simulink model "testScript_model_EGC"  (Simulink 8.1)
settings: Solver=ode3  SolverMode=SingleTasking  StartTime=0.0  StopTime=20000  FixedStep=Ts  RelTol=1e-3
PostLoadFcn:
  | Ts=1;
InitFcn:
  | Ts=1;
values from neighbouring files (symbols this model uses):
  CMD_signals = [0 300 600 900 1200 1500 1800 2100 2400 2700 3000 3300 ... (1568 elements, 49x32)]    [CMD_signals.mat]
libraries: artemis x1, rtio_generic_modbus x1, powerlib x1
settings Model: ARTEMISmethode_block_infos=$$__separator__$$testScript_model_EGC/ARTEMIS Guide$$__separator__$$  Creator=ma25949  LastModifiedBy=ed12083
settings OptimizationCC: BlockReduction=off  BooleanDataType=off  ExpressionDepthLimit=128
settings DebuggingCC: SaveWithParameterizedLinksMsg=none  SignalResolutionControl=TryResolveAllWithWarning  SolverPrmCheckMsg=none  MultiTaskDSMMsg=warning  MultiTaskCondExecSysMsg=none  FcnCallInpInsideContextMsg=EnableAllAsError  StrictBusMsg=None
settings HardwareCC: TargetUnknown=on
settings RTWCC: IncludeERTFirstTime=on
settings GRTTargetCC: CombineOutputUpdateFcns=on  GRTInterface=off

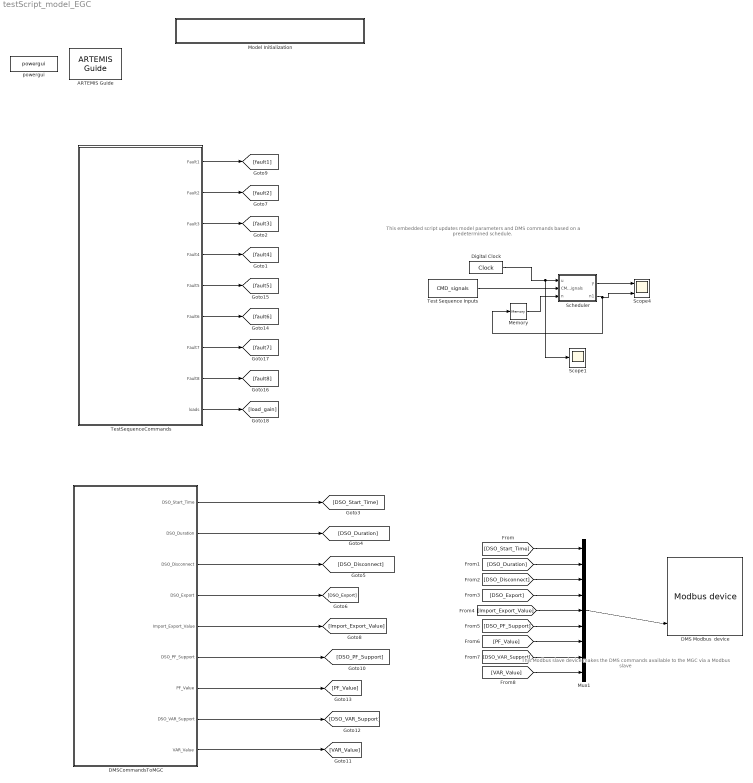
== system testScript_model_EGC ==
  note: This Modbus slave device makes the DMS
      | commands available to the MGC via a Modbus
      | slave
  note: This embedded script updates model
      | parameters and DMS commands based
      | on a predetermined schedule.
  ARTEMIS Guide : artemis/ARTEMIS/ARTEMIS Guide  Tag=FTSSmethode_opal_4hx0r99  Description=5.0_z1  lock=on  Ts=Ts  opt=art5  dyna=off  nb_perm=4  RT_fullcomp=off  ssn=on  ssn_itvc=off  ssn_ivic=off  ssn_ext=off  ssn_solver=Art5 with Backward Euler nodal interface  ssn_impulse=off  ssn_quasimpulse=off  ssn_impulse_loop=2  paraExtinctionThy=off  Thy_Impulse=on  dtc=Off  dtc_opt=normal  ao=on  simtype=off  ct_mac=off  lin_mov=off  lsp=[0.001 2]  spike_skip=Disabled  dtc_extra=1  dtc_sws=normal  dtc_pied=0.5  SPSRulesBlock=SPSRules  tre=on  ctmm=off  LF=off  dpl_type=ARTEMiS DPL  rlc_type=off  custom_type=off  para=on  ssn_ImpulseLoopBlockedStateUpdate=2  ssn_mov_iter_number=5  ssn_switch_iter_number=5
  DMS Modbus  device : rtio_generic_modbus/Modbus device  conf_name=DMS_slave_cfg.opal  conf_name_mask=DMS_slave_cfg.xls  sample_time=0
  DMSCommandsToMGC : Subsystem  mask{DSO_Start_Time=0, DSO_Duration=0, DSO_Disconnect=0, DSO_Export=0, Import_Export_Value=0, DSO_PF_Support=0, PF_Value=0, DSO_VAR_Support=0, VAR_Value=1000}
      mask prompts: DSO_Start_Time "DSO Start Time"; DSO_Duration "DSO Duration"; DSO_Disconnect "DSO Disconnect"; DSO_Export "DSO Export (1) or Import (0)"; Import_Export_Value "Import/Export Value, kW"; DSO_PF_Support "DSO PF Support (1) or Not (0)"; PF_Value "PF Value, pu, "+"(lagging) "-" (leading)"; DSO_VAR_Support "DSO VAR Support (1) or Not (0)"; VAR_Value "Import/Export Value, kVAr"
  Digital Clock : DigitalClock  SampleTime=Ts
  Memory : Memory  X0=1
  Model Initialization : Subsystem  AncestorBlock=artemis/Tools /Misc/Model Initialization  mask(Model Functions){InitFcnX=Ts=1;, prel=off, posl=on, inif=on, strf=off}
      mask prompts: InitFcnX "Initialisation"; prel "Preload Function"; posl "PostLoad Function"; inif "InitFcn"; strf "StartFcn"
      mask init:
      | currentBlock = gcb;
      | root = bdroot(currentBlock);
      | 
      | 
      | if ~strcmp(get_param(root,'BlockDiagramType'),'library')
      |     if prel==1
      |         set_param(root, 'PreLoadFcn', InitFcnX);
      |     else
      |         set_param(root, 'PreLoadFcn', '');
      |     end
      |     if inif==1
      |         set_param(root, 'InitFcn', InitFcnX);
      |     else
      |         set_param(root, 'InitFcn', '');
      |     end
      |     if strf==1
      |         set_param(root, 'StartFcn', InitFcnX);
      |     else
      |         set_param(root, 'StartFcn', '');
      |     end
      |     if posl==1
      |         set_param(root, 'PostLoadFcn', InitFcnX);
      |     else
      |         set_param(root, 'PostLoadFcn', '');
      |     end
      | end
      | 
      | pos = get_param(currentBlock, 'Position');
      | width = pos(3) - pos(1); height = pos(4) - pos(2);
      | txt = [ upper(root) '\n' '- InitFcn. . . . . '  get_param(root, 'InitFcn') ];
      settings: CopyFcn=set_param(gcb,'LinkStatus','inactive')
      mask Display: text(5, height*0.5, txt, 'horizontalAlignment', 'left', 'verticalAlignment', 'middle') ;
  Mux1 : Mux  Inputs=9
  Scheduler : MATLAB Function  TreatAsAtomicUnit=on
  Scope1 : Scope
      settings: YMin=1.04083e-17  YMax=0.2  SaveName=ScopeData4
  Scope4 : Scope  NumInputPorts=3
      settings: YMin=-5~-5~-5  YMax=5~5~5
  Test Sequence Inputs : Constant  Value=CMD_signals
  TestSequenceCommands : Subsystem  mask{fault1=0, fault2=0, fault3=0, fault4=0, fault5=0, fault6=0, fault7=0, fault8=0, load_gain=1}
      mask prompts: load_gain "Loads"
  powergui : powerlib/powergui  Priority=2  SimulationMode=Discrete  SolverType=Tustin  SampleTime=Ts  frequency=60  SPID=off  DisableSnubberDevices=off  DisableRonSwitches=off  DisableVfSwitches=off  SwTol=0  Interpol=off  DisplayEquations=off  frequencyindice=0  Pbase=100e6  ErrMax=1e-4  Iterations=50  UnitsV=kV  UnitsW=MW  FunctionMessages=off  echomessages=off  HookPort=off  EnableUseOfTLC=off  x0status=blocks  RestoreLinks=warning  ResistiveCurrentMeasurement=off  Frange=logspace(0,3,50)  Ylog=off  Xlog=off  ShowGrid=off  save=off  variable=ZData  structure=0  ZoomFFT=on  StartTime=0.0  cycles=2  DisplayStyle=off  fundamental=60  FreqAxis=off  MaxFrequency=1000  frequencyindicesteady=1  RmsSteady=1  display=off  Ts=0  methode=off
  wires:
  Mux1/1 -> DMS Modbus  device/4
  Scheduler/1(y) -> Scope4/1
  Scheduler/2(n1) -> Scope4/3, Memory/1
  Memory/1 -> Scheduler/3(n)
  Test Sequence Inputs/1 -> Scheduler/2(CMD_signals)
  Digital Clock/1 -> Scope1/1, Scheduler/1(u)
  DMSCommandsToMGC/3(DSO_Disconnect) -> [DSO_Disconnect]
  DMSCommandsToMGC/4(DSO_Export) -> [DSO_Export]
  DMSCommandsToMGC/6(DSO_PF_Support) -> [DSO_PF_Support]
  DMSCommandsToMGC/8(DSO_VAR_Support) -> [DSO_VAR_Support]
  DMSCommandsToMGC/9(VAR_Value) -> [VAR_Value]
  DMSCommandsToMGC/7(PF_Value) -> [PF_Value]
  DMSCommandsToMGC/1(DSO_Start_Time) -> [DSO_Start_Time]
  DMSCommandsToMGC/2(DSO_Duration) -> [DSO_Duration]
  DMSCommandsToMGC/5(Import_Export_Value) -> [Import_Export_Value]
  [DSO_Start_Time] -> Mux1/1
  [DSO_Duration] -> Mux1/2
  [DSO_Disconnect] -> Mux1/3
  [DSO_Export] -> Mux1/4
  [Import_Export_Value] -> Mux1/5
  [DSO_PF_Support] -> Mux1/6
  [PF_Value] -> Mux1/7
  [DSO_VAR_Support] -> Mux1/8
  [VAR_Value] -> Mux1/9
  TestSequenceCommands/1(Fault1) -> [fault1]
  TestSequenceCommands/2(Fault2) -> [fault2]
  TestSequenceCommands/3(Fault3) -> [fault3]
  TestSequenceCommands/4(Fault4) -> [fault4]
  TestSequenceCommands/5(Fault5) -> [fault5]
  TestSequenceCommands/6(Fault6) -> [fault6]
  TestSequenceCommands/7(Fault7) -> [fault7]
  TestSequenceCommands/8("Fault8 ") -> [fault8]
  TestSequenceCommands/9(loads) -> [load_gain]

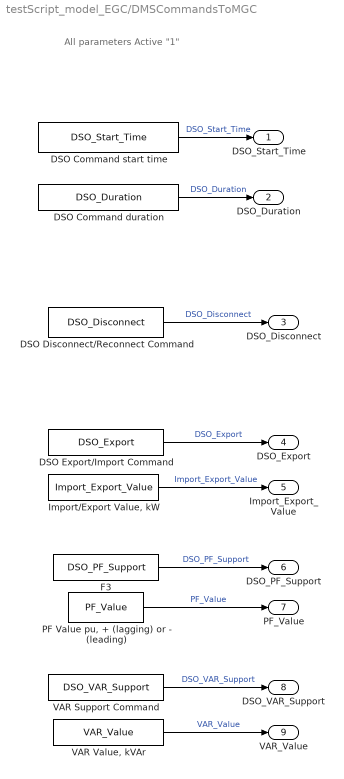
== system testScript_model_EGC/DMSCommandsToMGC ==
  note: All parameters Active "1"
  DSO Command duration : Constant  Value=DSO_Duration
  DSO Command start time : Constant  Value=DSO_Start_Time
  DSO Disconnect/Reconnect Command : Constant  Value=DSO_Disconnect
  DSO Export/Import Command : Constant  Value=DSO_Export
  F3 : Constant  Value=DSO_PF_Support
  "Import/Export Value, kW" : Constant  Value=Import_Export_Value
  "PF Value pu, + (lagging) or - (leading)" : Constant  Value=PF_Value
  VAR Support Command : Constant  Value=DSO_VAR_Support
  "VAR Value, kVAr" : Constant  Value=VAR_Value
  DSO_Start_Time : Outport
  DSO_Duration : Outport  Port=2
  DSO_Disconnect : Outport  Port=3
  DSO_Export : Outport  Port=4
  Import_Export_Value : Outport  Port=5
  DSO_PF_Support : Outport  Port=6
  PF_Value : Outport  Port=7
  DSO_VAR_Support : Outport  Port=8
  VAR_Value : Outport  Port=9
  wires:
  DSO Disconnect/Reconnect Command/1 -> DSO_Disconnect/1  "DSO_Disconnect"
  DSO Export/Import Command/1 -> DSO_Export/1  "DSO_Export"
  F3/1 -> DSO_PF_Support/1  "DSO_PF_Support"
  VAR Support Command/1 -> DSO_VAR_Support/1  "DSO_VAR_Support"
  "VAR Value, kVAr"/1 -> VAR_Value/1  "VAR_Value"
  "PF Value pu, + (lagging) or - (leading)"/1 -> PF_Value/1  "PF_Value"
  DSO Command start time/1 -> DSO_Start_Time/1  "DSO_Start_Time"
  DSO Command duration/1 -> DSO_Duration/1  "DSO_Duration"
  "Import/Export Value, kW"/1 -> Import_Export_Value/1  "Import_Export_Value"

== system testScript_model_EGC/Model Initialization ==

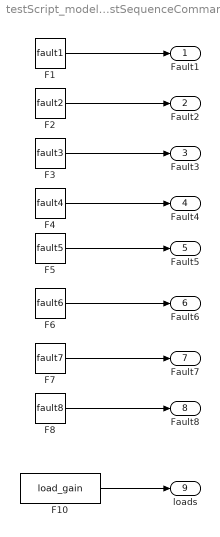
== system testScript_model_EGC/TestSequenceCommands ==
  F1 : Constant  Value=fault1
  F10 : Constant  Value=load_gain
  F2 : Constant  Value=fault2
  F3 : Constant  Value=fault3
  F4 : Constant  Value=fault4
  F5 : Constant  Value=fault5
  F6 : Constant  Value=fault6
  F7 : Constant  Value=fault7
  F8 : Constant  Value=fault8
  Fault1 : Outport
  Fault2 : Outport  Port=2
  Fault3 : Outport  Port=3
  Fault4 : Outport  Port=4
  Fault5 : Outport  Port=5
  Fault6 : Outport  Port=6
  Fault7 : Outport  Port=7
  "Fault8 " : Outport  Port=8
  loads : Outport  Port=9
  wires:
  F1/1 -> Fault1/1
  F2/1 -> Fault2/1
  F3/1 -> Fault3/1
  F4/1 -> Fault4/1
  F5/1 -> Fault5/1
  F8/1 -> "Fault8 "/1
  F6/1 -> Fault6/1
  F7/1 -> Fault7/1
  F10/1 -> loads/1

== matlab function Scheduler ==
  data: u input double; y output double; CMD_signals input double; n input double; n1 output double
function [y,n1] = fcn(u,CMD_signals,n)
% Author: Matthew Backes, MIT Lincoln Laboratory
% Date: 8/16/2016
%
% Edited 9/6/2016 by E. Corbett to remove repeated Modbus register 0007 for
% DSO Import value
%
% This function takes in the test sequence signals from a .mat file which
% is generated with the ____.m script. It then updates the parameters
% within the simulink model according to the time stamp of the test
% sequence command signals.
% CMD column 1 = time
% CMD column 2 = POI feeder 1 SEL relay
% CMD column 3 = POI feeder 2 SEL relay
% CMD column 4 = POI feeder 3 SEL relay
% CMD column 5 = diesel breaker
% CMD column 6 = solar irradiance gain
% CMD column 7 = solar breaker
% CMD column 8 = CHP breaker
% CMD column 9 = load gain
% CMD column 10 = motor 1 breaker
% CMD column 11 = motor 2 breaker
% CMD column 12 = fault location 1
% CMD column 13 = fault location 2
% CMD column 14 = fault location 3
% CMD column 15 = fault location 4
% CMD column 16 = fault location 5
% CMD column 17 = fault location 6
% CMD column 18 = fault location 7
% CMD column 19 = fault location 8 SECT
%
% Next section is for dso modbus slave
% 
% CMD column 20 = dso Disconnect command
% CMD column 21 = dso Reconnect command
% CMD column 22 = dso Export command
% CMD column 23 = dso Import command
% CMD column 24 = dso power factor command
% CMD column 25 = dso VAR support command
% CMD column 26 = dso Demand Response command
% CMD column 27 = dso Import/export value
% CMD column 28 = dso power factor value
% CMD column 29 = dso VAR value
% CMD column 30 = dso DR value
% CMD column 31 = dso Command start time
% CMD column 32 = dso command duration

y = u;

coder.extrinsic('set_param') %declare set_param as an extrinsic function
coder.extrinsic('num2str') %declare num2str as an extrinsic function
coder.extrinsic('tcpip')

time = CMD_signals(:,1); 
%time_lastCMD = time(length(time)); %do i need this anymore?
numCMDs = length(time);
DMS_ipaddr = '192.168.10.40';
%DMS_ipaddr = '127.0.0.1';
POI_F1_ipaddr = '192.168.10.41';
POI_F2_ipaddr = '192.168.10.42';
POI_F3_ipaddr = '192.168.10.43';
port = 512;

handles=tcpip(DMS_ipaddr, port,'Timeout',1);    %Create the tcpip object
set(handles, 'InputBufferSize', 512);       %assign the buffer
set(handles, 'ByteOrder', 'bigEndian');              %specify the order in which bytes are transmitted

% set(handles, 'Connected', 0);                            %default is not connected
% try 
Status=get(handles, 'Status');
%    if ~strcmp(Status,'open')       %if not open then 
%        Tcp=get(handles, 'tcp');
%%%%%%%%%%%        fopen(handles);                     %open a connection
%        set(handles, 'connected', 1);                   %connected
%    end


if n > numCMDs   %do nothing if we have exhausted all commands
    n1 = n;
else
    if u > time(n) % when the simulation time is greater than the command signal time, execute set_param
        n1 = n+1; % increment to next command to execute
        
        %parameters to set within simulink model
        set_param('testScript_model_EGC/TestSequenceCommands','load_gain',num2str(CMD_signals(n,9)),'fault1',num2str(CMD_signals(n,12)),'fault2',num2str(CMD_signals(n,13)),'fault3',num2str(CMD_signals(n,14)),'fault4',num2str(CMD_signals(n,15)),'fault5',num2str(CMD_signals(n,16)),'fault6',num2str(CMD_signals(n,17)),'fault7',num2str(CMD_signals(n,18)),'fault8',num2str(CMD_signals(n,19))); 
%%%
        set_param('testScript_model_EGC/DMSCommandsToMGC','DSO_Start_Time',num2str(CMD_signals(n,31)),'DSO_Duration',num2str(CMD_signals(n,32)),'DSO_Disconnect',num2str(CMD_signals(n,20)),'DSO_Export',num2str(CMD_signals(n,22)),'Import_Export_Value',num2str(CMD_signals(n,27)),'DSO_PF_Support',num2str(CMD_signals(n,24)),'PF_Value',num2str(CMD_signals(n,28)),'DSO_VAR_Support',num2str(CMD_signals(n,25)),'VAR_Value',num2str(CMD_signals(n,30)));
        
        
     else  % wait until the simulation time has eclisped the next command time
        n1 = n; 
    end
end
